simulink model "exp2_3"  (R2019a)
settings: Solver=VariableStepAuto  StartTime=0.0  StopTime=10000  RelTol=1e-3
libraries: simulink x1
settings Model: Creator=83621  LastModifiedBy=83621

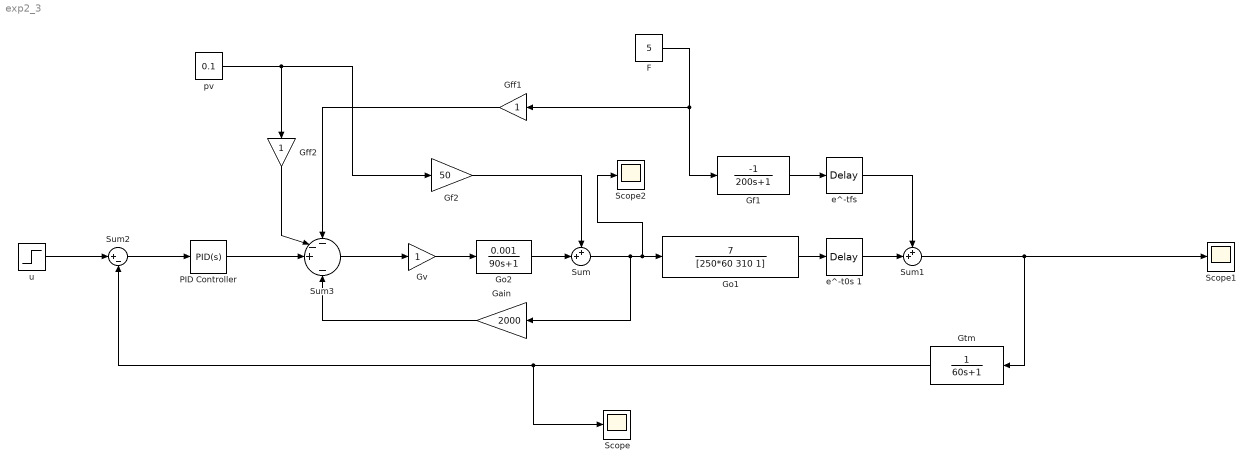
== system exp2_3 ==
  F : Constant  Value=5
  Gain : Gain  Gain=2000
  Gf1 : TransferFcn  Numerator=[-1]  Denominator=[200 1]
  Gf2 : Gain  Gain=50
  Gff1 : Gain
  Gff2 : Gain
  Go1 : TransferFcn  Numerator=[7]  Denominator=[250*60 310 1]
  Go2 : TransferFcn  Numerator=[0.001]  Denominator=[90 1]
  Gtm : TransferFcn  Denominator=[60 1]
  Gv : Gain
  PID Controller : simulink/Continuous/PID Controller  Controller=PID  Form=Parallel  TimeDomain=Continuous-time  SampleTime=-1  IntegratorMethod=Forward Euler  FilterMethod=Forward Euler  ControllerParametersSource=internal  P=0.4  I=0.2  D=5  UseFilter=on  N=100  TunerSelectOption=Transfer Function Based (PID Tuner App)  InitialConditionSource=internal  InitialConditionForIntegrator=0  InitialConditionForFilter=0  DifferentiatorICPrevScaledInput=0  ExternalReset=none  TrackingMode=off  Kt=1  LimitOutput=off  UpperSaturationLimit=inf  LowerSaturationLimit=-inf  LinearizeAsGain=on  AntiWindupMode=none  Kb=1  POutMin=[]  POutMax=[]  IOutMin=[]  IOutMax=[]  DOutMin=[]  DOutMax=[]  NOutMin=[]  NOutMax=[]  SumOutMin=[]  SumOutMax=[]  SaturationOutMin=[]  SaturationOutMax=[]  PParamMin=[]  PParamMax=[]  IParamMin=[]  IParamMax=[]  DParamMin=[]  DParamMax=[]  NParamMin=[]  NParamMax=[]  KbParamMin=[]  KbParamMax=[]  KtParamMin=[]  KtParamMax=[]  KbOutMin=[]  KbOutMax=[]  KtOutMin=[]  KtOutMax=[]  IntegratorOutMin=[]  IntegratorOutMax=[]  FilterOutMin=[]  FilterOutMax=[]  SumI1OutMin=[]  SumI1OutMax=[]  SumI2OutMin=[]  SumI2OutMax=[]  SumI3OutMin=[]  SumI3OutMax=[]  SumI4OutMin=[]  SumI4OutMax=[]  SumDOutMin=[]  SumDOutMax=[]  DifferentiatorOutMin=[]  DifferentiatorOutMax=[]  FilterDiffOutCoefMin=[]  FilterDiffOutCoefMax=[]  ReciprocalOutMin=[]  ReciprocalOutMax=[]  SumDenOutMin=[]  SumDenOutMax=[]  SumNumOutMin=[]  SumNumOutMax=[]  DivideOutMin=[]  DivideOutMax=[]  IntegratorContinuousStateAttributes=''  IntegratorStateMustResolveToSignalObject=off  IntegratorRTWStateStorageClass=Auto  FilterContinuousStateAttributes=''  FilterStateMustResolveToSignalObject=off  FilterRTWStateStorageClass=Auto  ParallelPVariant=InternalParameters  IdealPVariant=Disabled  IVariant=InternalParameters  DVariant=InternalParameters  IntegratorVariant=Continuous  SatVariant=Disabled  AWVariant=Passthrough  PCopyVariant=Disabled  TRVariant=Disabled  FdbkBlocksVariant=Forward  IdealPFdbkVariant=Disabled  SatFdbkVariant=Disabled  DerivativeFilterVariant=ContFilter  NVariant=InternalParameters  NCopyVariant=Disabled  FilterICVariant=InternalICsFilter  IntegratorICVariant=InternalICs  ExternalResetVariant=Disabled  TRSumVariant=Passthrough  SumFdbkVariant=Disabled  SumVariant=Sum_PID
  Scope : Scope
  Scope1 : Scope
  Scope2 : Scope
  Sum : Sum  Inputs=++|
  Sum1 : Sum  Inputs=++|
  Sum2 : Sum  Inputs=|+-
  Sum3 : Sum  Inputs=--+|-
  e^-t0s 1 : TransportDelay  DelayTime=120
  "e^-tfs " : TransportDelay  DelayTime=240
  pv : Constant  Value=0.1
  u : Step  After=5  SampleTime=0
  wires:
  pv/1 -> Gf2/1, Gff2/1
  Go2/1 -> Sum/2
  Sum/1 -> Gain/1, Scope2/1, Go1/1
  e^-t0s 1/1 -> Sum1/2
  Go1/1 -> e^-t0s 1/1
  Gf1/1 -> "e^-tfs "/1
  F/1 -> Gf1/1, Gff1/1
  Sum1/1 -> Scope1/1, Gtm/1
  u/1 -> Sum2/1
  Gtm/1 -> Scope/1, Sum2/2
  Gf2/1 -> Sum/1
  "e^-tfs "/1 -> Sum1/1
  Sum2/1 -> PID Controller/1
  Gv/1 -> Go2/1
  Sum3/1 -> Gv/1
  Gff2/1 -> Sum3/2
  PID Controller/1 -> Sum3/3
  Gff1/1 -> Sum3/1
  Gain/1 -> Sum3/4
